simulink model "NLI_B3"  (R2024a)
settings: Solver=FixedStepDiscrete  StartTime=0.0  StopTime=25  MaxStep=1/60  RelTol=1e-4  AbsTol=1e-3  EnableMultiTasking=on
PreLoadFcn:
  | Ts=100e-6;
undefined symbols (not defined in the file): D1, Delta
libraries: spsSequenceAnalyzerLib x4, spsThreePhaseVIMeasurementLib x3, spsGroundLib x2, spsThreePhaseSeriesRLCBranchLib x1, spsThreePhaseProgrammableVoltageSourceLib x1, spsThreePhaseParallelRLCLoadLib x1, spsThreePhaseMutualInductanceZ1Z0Lib x1, spsRMSLib x1, simulink x1, spsThreePhaseDynamicLoadLib x1, spsThreePhaseParallelRLCBranchLib x1, spsThreePhaseTapChangingTransformerTwoWindingsLib x1
settings Model: SimulationMode=accelerator  Creator=The MathWorks, Inc.  LastModifiedBy=VICTUS
settings SolverCC: AutoScaleAbsTol=off  AlgebraicLoopSolver=TrustRegion
settings DataIOCC: LimitDataPoints=on  SaveFormat=Array  ReturnWorkspaceOutputs=off  SignalLoggingName=sigsOut
settings OptimizationCC: ExpressionDepthLimit=2147483647  InitFltsAndDblsToZero=on  EfficientMapNaN2IntZero=off  LifeSpan=inf
settings DebuggingCC: SaveWithParameterizedLinksMsg=none  UnderspecifiedInitializationDetection=Classic  MergeDetectMultiDrivingBlocksExec=none  CheckExecutionContextPreStartOutputMsg=on  SignalResolutionControl=TryResolveAllWithWarning  MultiTaskDSMMsg=warning  MultiTaskCondExecSysMsg=none  FcnCallInpInsideContextMsg=warning  UnconnectedInputMsg=warning  UnconnectedOutputMsg=warning  UnconnectedLineMsg=warning  AllowSymbolicDim=off  StateNameClashWarn=warning  SFUnexpectedBacktrackingDiag=warning  SFNoUnconditionalDefaultTransitionDiag=warning  SFExecutionAtInitializationDiag=none  ArithmeticOperatorsInVariantConditions=warning
settings HardwareCC: ProdBitPerPointer=32  ProdBitPerSizeT=32  ProdBitPerPtrDiffT=32  ProdLargestAtomicFloat=None  ProdIntDivRoundTo=Undefined  ProdEndianess=Unspecified  ProdWordSize=32  ProdHWDeviceType=32-bit Generic  TargetUnknown=on
settings ModelReferenceCC: UpdateModelReferenceTargets=IfOutOfDate  EnableRefExpFcnMdlSchedulingChecks=on  PropagateSignalLabelsOutOfModel=off
settings SFSimCC: SimUseLocalCustomCode=off
settings RTWCC: RTWUseLocalCustomCode=off  GPUComputeCapability=3.5  DLArmComputeVersion=19.05
settings CodeAppCC: StateflowObjectComments=on
settings GRTTargetCC: TargetFcnLib=ansi_tfl_tmw.mat  TargetLangStandard=C89/C90 (ANSI)  CombineOutputUpdateFcns=off  GRTInterface=on
settings ConfigComp: CovMetricSettings=dw  CovSaveCumulativeToWorkspaceVar=on  CovSaveSingleToWorkspaceVar=on  CovExternalEMLEnable=off  CovSFcnEnable=off
settings SimscapeCC: SimscapeNormalizeSystem=off

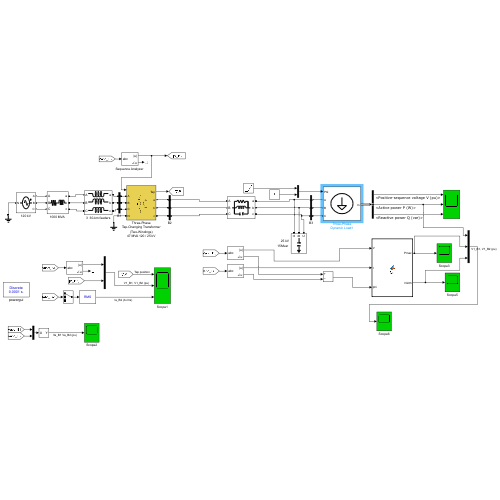
[thumbnail: Simulink's stored preview of the top-level diagram]
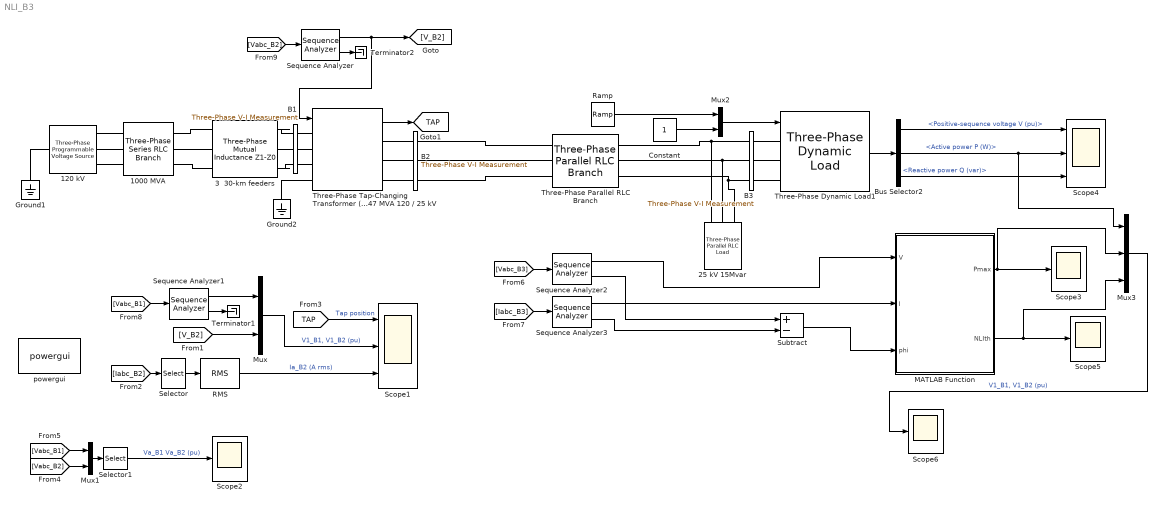
== system NLI_B3 ==
  "1000 MVA " : spsThreePhaseSeriesRLCBranchLib/Three-Phase Series RLC Branch  LConnTagsString=A|B|C  RConnTagsString=A|B|C  BranchType=RL  Resistance=120e3^2/1000e6/10  Inductance=120e3^2/1000e6/(2*pi*60)  Capacitance=1.0  Measurements=None
  120 kV : spsThreePhaseProgrammableVoltageSourceLib/Three-Phase Programmable Voltage Source  PositiveSequence=[120e3 0 60]  VariationEntity=Amplitude  VariationType=Table of time-amplitude pairs  VariationTypeAlt=Step  VariationStep=0.2  VariationRate=10  VariationMagnitude=0.3  VariationFrequency=2  VariationTiming="[5  20]"  VariationPhaseA=off  Amplitudes="[ 1  1  1 ]"  TimeValues="[0  2  10]"  HarmonicGeneration=off  HarmonicA=[3 0.2 -25 0]  HarmonicB=[2 0.15 35 2]  Timing="[0.05  3]"  BusType=PV  Pref=2.234  Qref=0  Qmin=0  Qmax=2
  "25 kV 15Mvar " : spsThreePhaseParallelRLCLoadLib/Three-Phase Parallel RLC Load  LConnTagsString=A|B|C  Configuration=Y (grounded)  NominalVoltage=25e3  Vabc=[1e3 1e3 1e3]  Vabcp=[1e3 1e3 1e3]  NominalFrequency=60  UnbalancedPower=off  ActivePower=0  InductivePower=0  CapacitivePower=15e6  Pabc=[10e3 9e3 11e3]  QLabc=[100 90 110]  QCabc=[100 90 110]  Pabcp=[10e3 9e3 11e3]  QLabcp=[100 90 110]  QCabcp=[100 90 110]  Measurements=None  LoadType=constant Z
  3  30-km feeders : spsThreePhaseMutualInductanceZ1Z0Lib/Three-Phase Mutual Inductance Z1-Z0  LConnTagsString=a|b|c  RConnTagsString=A|B|C  PositiveSequence=[ 0.1153 , 1.048e-3 ]*30/3  ZeroSequence=[ 0.4130 , 3.321e-3 ]*30/3
      settings: AttributesFormatString=\n
  B1 : spsThreePhaseVIMeasurementLib/Three-Phase V-I Measurement  VoltageMeasurement=phase-to-ground  SetLabelV=on  LabelV=Vabc_B1  Vpu=on  VpuLL=off  CurrentMeasurement=no  SetLabelI=on  LabelI=IabcB3  Ipu=on  Pbase=47e6  Vbase=120e3  OutputType=Complex  PhasorSimulation=off  PSBequivalent=0
  B2 : spsThreePhaseVIMeasurementLib/Three-Phase V-I Measurement  VoltageMeasurement=phase-to-ground  SetLabelV=on  LabelV=Vabc_B2  Vpu=on  VpuLL=off  CurrentMeasurement=yes  SetLabelI=on  LabelI=Iabc_B2  Ipu=off  Pbase=47e6  Vbase=25e3  OutputType=Complex  PhasorSimulation=off  PSBequivalent=0
  B3 : spsThreePhaseVIMeasurementLib/Three-Phase V-I Measurement  VoltageMeasurement=phase-to-ground  SetLabelV=on  LabelV=Vabc_B3  Vpu=on  VpuLL=off  CurrentMeasurement=yes  SetLabelI=on  LabelI=Iabc_B3  Ipu=off  Pbase=47e6  Vbase=25e3  OutputType=Complex  PhasorSimulation=off  PSBequivalent=0
  Bus Selector2 : BusSelector  OutputSignals=Positive-sequence voltage V (pu),Active power P (W),Reactive power Q (var)
  Constant : Constant
  Ground1 : spsGroundLib/Ground  LConnTagsString=a
  Ground2 : spsGroundLib/Ground  LConnTagsString=a
  MATLAB Function : MATLAB Function  TreatAsAtomicUnit=on
  Mux : Mux  Inputs=2
  Mux1 : Mux  Inputs=2
  Mux2 : Mux  Inputs=2
  Mux3 : Mux  Inputs=3
  RMS : spsRMSLib/RMS  TrueRMS=on  Freq=60  RMSInit=0  Ts=Ts
  Ramp : simulink/Sources/Ramp  slope=1  start=0  InitialOutput=0
  Scope1 : Scope  NumInputPorts=3
  Scope{2..3,5..6} (4 alike) : Scope
  Scope4 : Scope  NumInputPorts=3
  Selector : Selector  InputPortWidth=3  IndexOptions=Index vector (dialog)  Indices=1  OutputSizes=1
  Selector1 : Selector  InputPortWidth=6  IndexOptions=Index vector (dialog)  Indices=[1 4]  OutputSizes=1
  "Sequence Analyzer " : spsSequenceAnalyzerLib/Sequence Analyzer  Freq=60  n=1  seq=Positive  InInit=[1, 0]  Ts=Ts
  Sequence Analyzer1 : spsSequenceAnalyzerLib/Sequence Analyzer  Freq=60  n=1  seq=Positive  InInit=[1, 0]  Ts=Ts
  Sequence Analyzer2 : spsSequenceAnalyzerLib/Sequence Analyzer  Freq=60  n=1  seq=Positive  InInit=[1, 0]  Ts=Ts
  Sequence Analyzer3 : spsSequenceAnalyzerLib/Sequence Analyzer  Freq=60  n=1  seq=Positive  InInit=[1, 0]  Ts=Ts
  Subtract : Sum  Inputs=+-
  Terminator1 : Terminator
  Terminator2 : Terminator
  Three-Phase Dynamic Load1 : spsThreePhaseDynamicLoadLib/Three-Phase Dynamic Load  NominalVoltage=[ 25e3 60 ]  ActiveReactivePowers=[0 10e6]  PositiveSequence=[1 0]  ExternalControl=on  NpNq=[1.3 2]  TimeConstants="[0  0  0  0]"  MinimumVoltage=0.7  Tfilter=1e-4  LoadFlowParameters=[4,0,0,0,0]
      settings: LibrarySourceBlock=|
      | sps_lib/Passives/Three-Phase
      | Dynamic Load
  Three-Phase Parallel RLC Branch : spsThreePhaseParallelRLCBranchLib/Three-Phase Parallel RLC Branch  LConnTagsString=A|B|C  RConnTagsString=A|B|C  BranchType=RLC  Resistance=1e6  Inductance=1e-3  Capacitance=0  Measurements=None
  Three-Phase Tap-Changing Transformer (Two-Windings) 47 MVA 120 / 25 kV : spsThreePhaseTapChangingTransformerTwoWindingsLib/Three-Phase Tap-Changing Transformer (Two-Windings)  NominalParameters=[ 47e6 , 60]  Winding1=[ 120e3 , 0.003 , 0.09 ]  Winding2Connection=Delta (D1)  Winding2=[ 25e3 , 0.003 , 0.09 ]  CoreType=Three-limb core (core-type)  L0=0.5  Rmag=300  Lmag=300  SetSaturation=off  SaturationCurrentFlux=[0 0; 0.002 1.0; 0.006 1.12; 0.009 1.15; 0.015 1.17; 0.03 1.19; 0.05 1.20; 0.08 1.21; 1.0 1.302]  SpecifyInitialFluxes=on  InitialFluxes=[ -1.0 0.5 0.5]  Measurements=None  MinTap=-16  MaxTap=+16  InitialTap=0  VoltageStep=0.00625  TapSelectionTime=5  ControlMode=Voltage regulation  Threshold=0.5  ReferenceVoltage=1.04  DeadBand=0.005  Delay=5
  powergui : spspowerguiLib/powergui  Priority=2  SimulationMode=Discrete  SampleTime=Ts  frequency=60  Iterations=50  frequencyindice=0  Pbase=100e6  ErrMax=1e-4  UnitsV=kV  UnitsW=MW  buscounter=0  FunctionMessages=off  echomessages=off  EnableUseOfTLC=off  CurrentSourceSwitches=off  DisableSnubberDevices=off  DisableRonSwitches=off  DisableVfSwitches=off  DisplayEquations=off  AutomaticDiscreteSolvers=on  SolverType=Tustin/Backward Euler (TBE)  Interpol=off  ExternalGateDelay=off  methode=off  Ts=0  x0status=blocks  SPID=off  SwTol=0  HookPort=off  NonlinearTolerance=1e-4  nMaxIteration=100  ContinueOnMaxIteration=off  RestoreLinks=warning  ResistiveCurrentMeasurement=off  Frange=[0:2:500]  Ylog=off  Xlog=on  ShowGrid=off  save=off  variable=ZData  structure=0  ZoomFFT=on  StartTime=0.0  cycles=1  DisplayStyle=1  fundamental=60  FreqAxis=off  MaxFrequency=1000  frequencyindicesteady=1  RmsSteady=2  display=off
  tag scope: TAP=global
  wires:
  [TAP] -> Scope1/1  "Tap position"
  Three-Phase Tap-Changing Transformer (Two-Windings) 47 MVA 120 / 25 kV/1 -> [TAP]
  "Sequence Analyzer "/1 -> Three-Phase Tap-Changing Transformer (Two-Windings) 47 MVA 120 / 25 kV/1, [V_B2]
  Sequence Analyzer1/1 -> Mux/1
  [Vabc_B2] -> "Sequence Analyzer "/1
  "Sequence Analyzer "/2 -> Terminator2/1
  Sequence Analyzer1/2 -> Terminator1/1
  [Vabc_B1] -> Sequence Analyzer1/1
  Mux/1 -> Scope1/2  "V1_B1, V1_B2 (pu)"
  [V_B2] -> Mux/2
  [Iabc_B2] -> Selector/1
  Selector/1 -> RMS/1
  RMS/1 -> Scope1/3  "Ia_B2 (A rms)"
  Selector1/1 -> Scope2/1  "Va_B1 Va_B2 (pu)"
  [Vabc_B2] -> Mux1/2
  Mux1/1 -> Selector1/1
  [Vabc_B1] -> Mux1/1
  Bus Selector2/1 -> Scope4/1  "<Positive-sequence voltage V (pu)>"
  Ramp/1 -> Mux2/1
  Bus Selector2/3 -> Scope4/3  "<Reactive power Q (var)>"
  Mux2/1 -> Three-Phase Dynamic Load1/1
  Bus Selector2/2 -> Mux3/1, Scope4/2  "<Active power P (W)>"
  Three-Phase Dynamic Load1/1 -> Bus Selector2/1
  Constant/1 -> Mux2/2
  Sequence Analyzer2/2 -> Subtract/1
  [Vabc_B3] -> Sequence Analyzer2/1
  Sequence Analyzer2/1 -> MATLAB Function/1(V)
  [Iabc_B3] -> Sequence Analyzer3/1
  Sequence Analyzer3/1 -> MATLAB Function/2(I)
  Sequence Analyzer3/2 -> Subtract/2
  Subtract/1 -> MATLAB Function/3(phi)
  MATLAB Function/1(Pmax) -> Mux3/2, Scope3/1
  MATLAB Function/2(NLIth) -> Mux3/3, Scope5/1
  Mux3/1 -> Scope6/1  "V1_B1, V1_B2 (pu)"
  connections:
  Three-Phase Tap-Changing Transformer (Two-Windings) 47 MVA 120 / 25 kV/LConn1 -- B1/RConn1
  Three-Phase Tap-Changing Transformer (Two-Windings) 47 MVA 120 / 25 kV/RConn3 -- B2/LConn3
  Ground1/LConn1 -- 120 kV/LConn1
  Three-Phase Tap-Changing Transformer (Two-Windings) 47 MVA 120 / 25 kV/RConn1 -- B2/LConn1
  Three-Phase Tap-Changing Transformer (Two-Windings) 47 MVA 120 / 25 kV/LConn2 -- B1/RConn2
  Three-Phase Tap-Changing Transformer (Two-Windings) 47 MVA 120 / 25 kV/RConn2 -- B2/LConn2
  120 kV/RConn2 -- "1000 MVA "/LConn2
  Three-Phase Tap-Changing Transformer (Two-Windings) 47 MVA 120 / 25 kV/LConn3 -- B1/RConn3
  120 kV/RConn3 -- "1000 MVA "/LConn3
  120 kV/RConn1 -- "1000 MVA "/LConn1
  Ground2/LConn1 -- Three-Phase Tap-Changing Transformer (Two-Windings) 47 MVA 120 / 25 kV/LConn4
  Three-Phase Parallel RLC Branch/RConn2 -- B3/LConn2 -- "25 kV 15Mvar "/LConn2
  "25 kV 15Mvar "/LConn1 -- B3/LConn1 -- Three-Phase Parallel RLC Branch/RConn1
  Three-Phase Parallel RLC Branch/RConn3 -- "25 kV 15Mvar "/LConn3 -- B3/LConn3
  B2/RConn1 -- Three-Phase Parallel RLC Branch/LConn1
  B2/RConn2 -- Three-Phase Parallel RLC Branch/LConn2
  B2/RConn3 -- Three-Phase Parallel RLC Branch/LConn3
  3  30-km feeders/RConn1 -- B1/LConn1
  3  30-km feeders/RConn2 -- B1/LConn2
  3  30-km feeders/RConn3 -- B1/LConn3
  "1000 MVA "/RConn1 -- 3  30-km feeders/LConn1
  "1000 MVA "/RConn2 -- 3  30-km feeders/LConn2
  "1000 MVA "/RConn3 -- 3  30-km feeders/LConn3
  B3/RConn1 -- Three-Phase Dynamic Load1/LConn1
  B3/RConn2 -- Three-Phase Dynamic Load1/LConn2
  B3/RConn3 -- Three-Phase Dynamic Load1/LConn3

== matlab function NLI_B3/MATLAB Function ==
  data: V input; Pmax output; I input; phi input; NLIth output
function [Pmax, NLIth] = fcn(V, I, phi)
    % Persistent variables to store previous values
    persistent V_prev I_prev phi_prev isFirstRun

    % Initialize on first run
    if isempty(isFirstRun)
        V_prev = 0;
        I_prev = 0;
        phi_prev = 0;
        isFirstRun = true;
    end

    % Step 1: Initialize lambda
    lambda = 1;

    % Step 2: Calculate Active and Reactive Power
    PL = V * I * cos(phi);
    QL = V * I * sin(phi);

    PL_prev = V_prev * I_prev * cos(phi_prev);
    QL_prev = V_prev * I_prev * sin(phi_prev);

    % Step 3: Calculate ZL^2 (Current and Previous)
    if I ~= 0
        ZL_sq = V^2 / I^2;
    else
        ZL_sq = 1e-6; % Safe default
    end

    if I_prev ~= 0
        ZL_prev_sq = V_prev^2 / I_prev^2;
    else
        ZL_prev_sq = 1e-6; % Safe default
    end

    % Step 4: Calculate RL, XL (Current and Previous)
    RL = (PL * ZL_sq) / (V^2 + 1e-6);
    XL = (QL * ZL_sq) / (V^2 + 1e-6);

    RL_prev = (PL_prev * ZL_prev_sq) / (V_prev^2 + 1e-6);
    XL_prev = (QL_prev * ZL_prev_sq) / (V_prev^2 + 1e-6);

    % Step 5: Calculate ZL, ZL_prev
    ZL = sqrt(RL^2 + XL^2);
    ZL_prev = sqrt(RL_prev^2 + XL_prev^2);

    % Step 6: Conductance GL, GL_prev
    GL = cos(phi) / (ZL + 1e-6);
    GL_prev = cos(phi_prev) / (ZL_prev + 1e-6);

    % Step 7: Update lambda from past data
    if abs(GL - GL_prev) > 1e-6
        lambda = (PL - PL_prev) / (GL - GL_prev);
    end

    % Step 8: Solve for Zth numerically using quadratic equation
    cos_phi_sq = cos(phi)^2;
    a = GL^2 * (lambda * GL^2 + I^2 * cos_phi_sq);
    b = 2 * lambda * GL^3 * cos(phi) * cos(phi);
    c = cos_phi_sq * (lambda * GL^2 - I^2 * cos_phi_sq);

    % Discriminant
    discrim = b^2 - 4 * a * c;

    if discrim >= 0 && a ~= 0
        root1 = (-b + sqrt(discrim)) / (2 * a);
        root2 = (-b - sqrt(discrim)) / (2 * a);
        Zth_candidate = max(root1, root2); % Pick positive real root
        if Zth_candidate > 0
            Zth = Zth_candidate;
        else
            Zth = 1; % Safe fallback
        end
    else
        Zth = 1; % Safe fallback
    end

    % Step 9: Solve for Eth using power formula
    denom_Eth = GL * cos_phi_sq + 1e-6;
    numerator = PL * (GL^2 * Zth^2 + 2 * GL * Zth * cos_phi_sq + cos_phi_sq);
    Eth_sq = numerator / denom_Eth;

    if Eth_sq < 0
        Eth = 0;
    else
        Eth = sqrt(Eth_sq);
    end

    % Step 10: Calculate alpha, gamma
    alpha = atan(XL / (RL + 1e-6));
    gamma = phi - alpha;

    % Step 11: Calculate Pmax
    denom_Pmax = 2 * Zth * (1 + cos(gamma)) + 1e-6;
    Pmax = (Eth^2 * cos(phi)) / denom_Pmax;

    % Step 12: Calculate NLIth
    NLIth = Zth / (ZL + 1e-6);

    % Update persistent values for next cycle
    V_prev = V;
    I_prev = I;
    phi_prev = phi;

    % Optional Debugging Outputs:
    % disp(['PL = ', num2str(PL), ', GL = ', num2str(GL), ', Zth = ', num2str(Zth), ', Eth = ', num2str(Eth), ', Pmax = ', num2str(Pmax)]);
end
